simulink model "addtest"  (R2020a)
settings: Solver=VariableStepAuto  StartTime=0.0  StopTime=10.0  RelTol=1e-3
libraries: roblocks x3
settings Model: Creator=93548  LastModifiedBy=93548

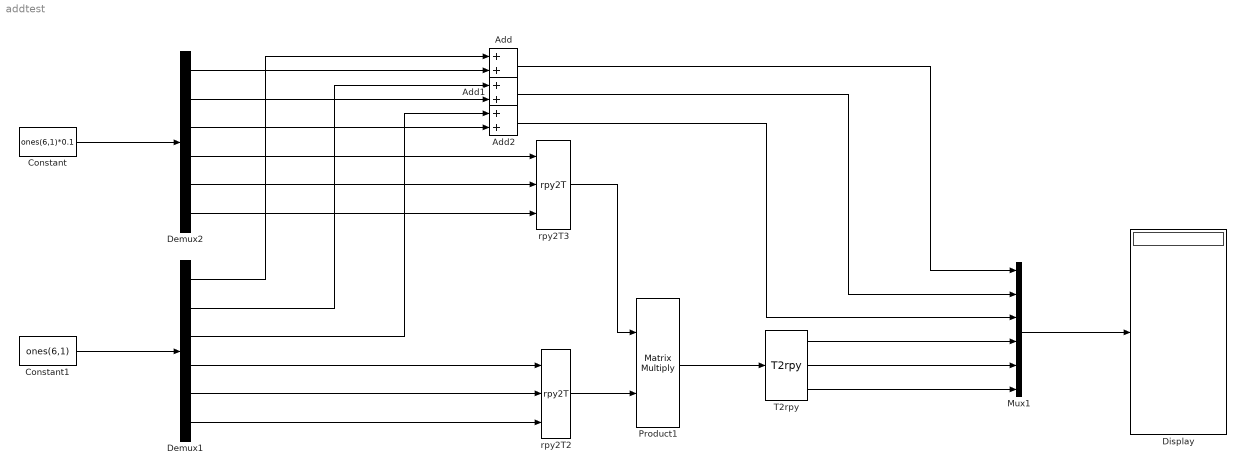
== system addtest ==
  Add : Sum
  Add1 : Sum
  Add2 : Sum
  Constant : Constant  Value=ones(6,1)*0.1
  Constant1 : Constant  Value=ones(6,1)
  Demux1 : Demux  Outputs=6
  Demux2 : Demux  Outputs=6
  Display : Display
  Mux1 : Mux  Inputs=6
  Product1 : Product  Multiplication=Matrix(*)
  T2rpy : roblocks/Toolbox/T2rpy  sequence=XYZ  degrees=off
  rpy2T2 : roblocks/Toolbox/rpy2T  sequence=XYZ  degrees=off
  rpy2T3 : roblocks/Toolbox/rpy2T  sequence=XYZ  degrees=off
  wires:
  Product1/1 -> T2rpy/1
  Demux2/5 -> rpy2T3/2
  rpy2T2/1 -> Product1/2
  Demux1/4 -> rpy2T2/1
  Add2/1 -> Mux1/3
  T2rpy/1 -> Mux1/4
  T2rpy/3 -> Mux1/6
  Demux1/2 -> Add1/1
  Demux1/5 -> rpy2T2/2
  Add/1 -> Mux1/1
  Demux2/2 -> Add1/2
  Mux1/1 -> Display/1
  Demux1/6 -> rpy2T2/3
  Demux1/1 -> Add/1
  Demux1/3 -> Add2/1
  Constant/1 -> Demux2/1
  Demux2/3 -> Add2/2
  Demux2/4 -> rpy2T3/1
  Add1/1 -> Mux1/2
  Demux2/1 -> Add/2
  Constant1/1 -> Demux1/1
  Demux2/6 -> rpy2T3/3
  T2rpy/2 -> Mux1/5
  rpy2T3/1 -> Product1/1
